simulink model "sarkac_RL"  (R2019b)
settings: Solver=ode45  StartTime=0.0  StopTime=2  FixedStep=1/1000  RelTol=1e-4  AbsTol=1e-4
libraries: vrlib x1
settings Model: SimulationMode=accelerator  EnablePacing=on  Creator=Fatabi  LastModifiedBy=Fatabi
settings SolverCC: ZeroCrossAlgorithm=Adaptive

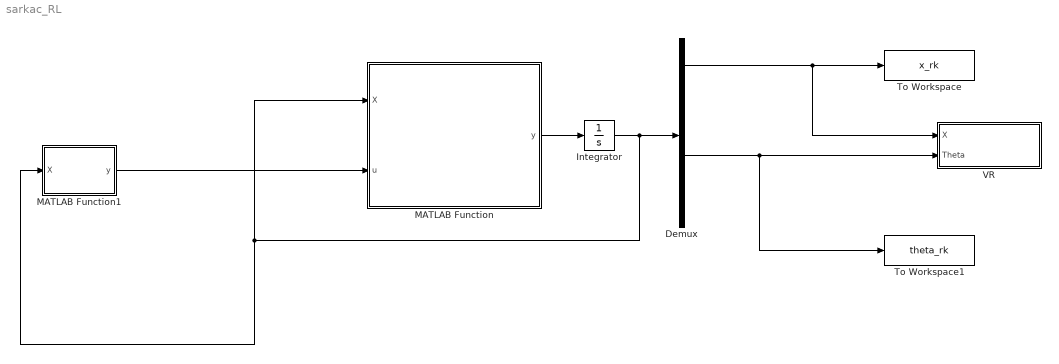
== system sarkac_RL ==
  Demux : Demux
  Integrator : Integrator  InitialCondition=[0,0,3*pi/4,0]
  MATLAB Function : MATLAB Function  TreatAsAtomicUnit=on
  MATLAB Function1 : MATLAB Function  TreatAsAtomicUnit=on
  To Workspace : ToWorkspace  VariableName=x_rk  SaveFormat=Timeseries  SampleTime=-1
  To Workspace1 : ToWorkspace  VariableName=theta_rk  SaveFormat=Timeseries  SampleTime=-1
  VR : Subsystem
  wires:
  MATLAB Function/1(y) -> Integrator/1
  Demux/3 -> To Workspace1/1, VR/2(Theta)
  Demux/1 -> VR/1("X "), To Workspace/1
  Integrator/1 -> MATLAB Function1/1(X), MATLAB Function/1(X), Demux/1
  MATLAB Function1/1(y) -> MATLAB Function/2(u)

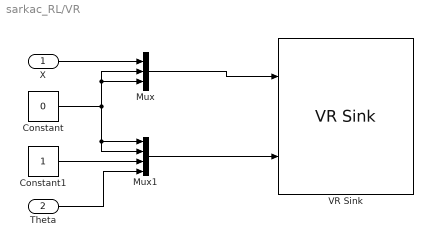
== system sarkac_RL/VR ==
  "X " : Inport
  Theta : Inport  Port=2
  Constant : Constant  Value=0
  Constant1 : Constant
  Mux : Mux  Inputs=3
  Mux1 : Mux
  VR Sink : vrlib/VR Sink  InstantiateOnLoad=on  SampleTime=0.05  ViewEnable=on  RemoteChange=off  RemoteView=off  FieldsWritten=Cart.translation.3.1.1.double#Pendulum.rotation.4.1.1.double  WorldFileName=Cart_Pendulum.wrl  AutoView=off  VideoDimensions=[]  AllowVariableSize=off
      settings: SourceProductName=Simulink
  wires:
  "X "/1 -> Mux/1
  Theta/1 -> Mux1/4
  Constant1/1 -> Mux1/3
  Constant/1 -> Mux1/2, Mux1/1, Mux/2, Mux/3
  Mux/1 -> VR Sink/1
  Mux1/1 -> VR Sink/2

== matlab function sarkac_RL/MATLAB Function1 ==
  settings: updateMethod=DISCRETE
  data: X input; y output
function y = fcn(X)
persistent layer1_w layer1_b layer2_w layer2_b 
if isempty(layer1_w)
layer1_w = randn(4,16);
layer1_b = randn(1,16);
layer2_w = randn(16,1);
layer2_b = randn(1,1);
end
X    = X';
out1 = X*layer1_w + layer1_b;
% activation1 = tanh(out1);
out2 = out1*layer2_w + layer2_b;
act2 = 100*(out2/(1+abs(out2)));
y = act2 ;
end

== matlab function sarkac_RL/MATLAB Function ==
  data: X input; u input; y output
function y = fcn(X,u)

M = .5;
m = 0.2;
d = 0.1;
% I = 0.006;
g = 9.8;
L = 0.3;

y = zeros(4,1);

I = 4/3*m*L^2;

% D = m*L*L*(M+m*(1-cos(x(3))^2));
% dx(1,1) = x(2);
% dx(2,1) = (1/D)*(m^2*L^2*g*cos(x(3))*sin(x(3)) + m*L^2*(m*L*x(4)^2*sin(x(3)) - d*x(2))) + m*L*L*(1/D)*u;
% dx(3,1) = x(4);
% dx(4,1) = (1/D)*(-(m+M)*m*g*L*sin(x(3)) - m*L*cos(x(3))*(m*L*x(4)^2*sin(x(3)) - d*x(2))) - m*L*cos(x(3))*(1/D)*u;

y(1,1) = X(2);
y(2,1) = (L^2*g*m^2*sin(2*X(3))/2 + (I + L^2*m)*(L*m*X(4)^2*sin(X(3)) - d*X(2) + u))/(-L^2*m^2*cos(X(3))^2 + (I + L^2*m)*(M + m));
y(3,1) = X(4);
y(4,1) = -m*L/(I + m*L^2) * (y(2,1)*cos(X(3)) + g*sin(X(3)));

% integral of theta error
% if nargin == 8
%     y(5,1) = x(3) - wr(3);
% end
end
